simulink model "stateAction"  (R2023b)
settings: Solver=FixedStepDiscrete  StartTime=0.0  StopTime=10.0  FixedStep=0.1  RelTol=1e-3  EnableMultiTasking=on
settings Model: Creator=NITRO  LastModifiedBy=NITRO
settings SolverCC: AlgebraicLoopSolver=TrustRegion  AutoInsertRateTranBlk=on
settings DataIOCC: LimitDataPoints=on
settings OptimizationCC: LifeSpan=inf
settings DebuggingCC: UnconnectedInputMsg=warning  UnconnectedOutputMsg=warning  UnconnectedLineMsg=warning  AllowSymbolicDim=off  SFUnexpectedBacktrackingDiag=warning  SFNoUnconditionalDefaultTransitionDiag=warning  SFExecutionAtInitializationDiag=none  ArithmeticOperatorsInVariantConditions=warning
settings ModelReferenceCC: EnableRefExpFcnMdlSchedulingChecks=on
settings SFSimCC: SimUseLocalCustomCode=off  CustomCodeUndefinedFunction=UseInterfaceOnly
settings RTWCC: RTWUseLocalCustomCode=off  DLArmComputeVersion=19.05
settings CodeAppCC: StateflowObjectComments=on
settings GRTTargetCC: TargetLangStandard=C89/C90 (ANSI)
settings ConfigComp: CovMetricSettings=dw  CovSaveCumulativeToWorkspaceVar=on  CovSaveSingleToWorkspaceVar=on  CovExternalEMLEnable=off  CovSFcnEnable=off

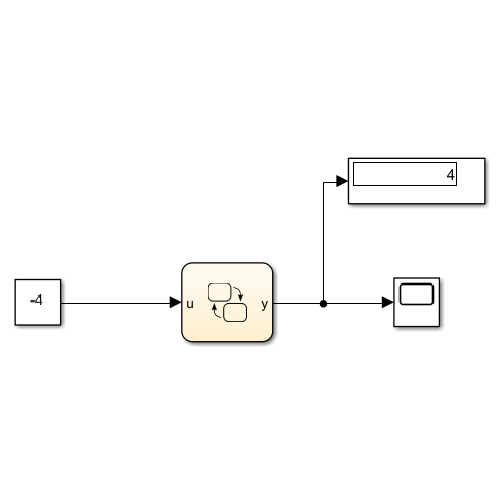
[thumbnail: Simulink's stored preview of the top-level diagram]
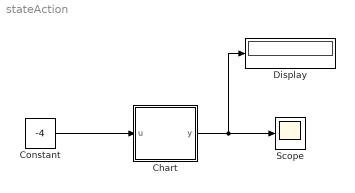
== system stateAction ==
  Chart : Stateflow chart  TreatAsAtomicUnit=on
  Constant : Constant  Value=-4
  Display : Display
  Scope : Scope
  wires:
  Constant/1 -> Chart/1(u)
  Chart/1(y) -> Display/1, Scope/1

== stateflow chart stateAction/Chart ==
  state A
    entry: y=3;
  state B
    entry: y=u+1;
    during: y=u;
    exit: y=-u;
  state C
    entry: y=0;
    exit: y=10;
  state D
  state E
  (default) -> A
  A -> B [order 1] : [u<=0]
  A -> C [order 2] : [u>0]
  B -> D : after(3,sec)
  C -> E : after(1,sec)
  data: u input; y output
